simulink model "flight_data_collection"  (R2024a)
settings: Solver=FixedStepAuto  StartTime=0.0  StopTime=inf  FixedStep=0.1
model workspace (MAT data in the model file):
  Ixx_values = 1.545e-05
  Iyy_values = 0.00073574
  Izz_values = 0.00074861
  base_link_Ixx = 7.46
  base_link_Iyy = 1.52
  base_link_Izz = 8.88
  base_link_mass = 19.0939
  gps0_Ixx = 2.1733e-06
  gps0_Iyy = 2.1733e-06
  gps0_Izz = 1.8e-07
  gps0_mass = 0.01
  i = 8
  imu_link_Ixx = 1e-05
  imu_link_Iyy = 1e-05
  imu_link_Izz = 1e-05
  imu_link_mass = 0.015
  masses = 0.085251
  phi = sym
  phi.s = 'symobj::fromString("eJytVL1OwzAQdpqWPwkhoaJCp0jwBIydCoKBEYoYWCyHmGLkOCXnlGbjKXgneCpst6LONQ0MjfTJzt35u+/uLIeEkBYhH59mbYdBxyzDPpl/odl3F3sTQ3YtoAQGIMbKmSv+c4t3LvIkmrJcsFjySLGUQ1QATyKhIijTLH69KtK0vEm40uJZ8Jz4OVuIs23xksnE2HteTL9mj/W6syAzjexbFqATKWKXe48sv30L4HpUphdSMOAwr/PEy/HtxQeIe9tiAoI+MFvY8MzTebo84/79vAcWc02DwfVskpmO4Vl8efFt9N9BfE6Hx+P7QgujEfOv1EF/J13xHVmsHeWSs1M7jyIGpP2wQYebFeVvBZPkr3429crn3LGATE65uwGV3jjfJQPxNOIa8fRQrKsn51ZZhd/hjlZ6gTV1US2+77hulkJpPnYdXs31uLlcrv6caZGp+rpu6eYejP9epKZHofniCJXw2UpeVyQ1iZkC6j0sliP0mhFEixXbgzX2+8X6AxDlhOk=", 2)'
  phi.Digits = 32
  rotors(1).mass = 0.085251
  rotors(1).Ixx = 1.545e-05
  rotors(1).Iyy = 0.00073574
  rotors(1).Izz = 0.00074861
  rotors(2).mass = 0.085251
  rotors(2).Ixx = 1.545e-05
  rotors(2).Iyy = 0.00073574
  rotors(2).Izz = 0.00074861
  rotors(3).mass = 0.085251
  rotors(3).Ixx = 1.545e-05
  rotors(3).Iyy = 0.00073574
  rotors(3).Izz = 0.00074861
  rotors(4).mass = 0.085251
  rotors(4).Ixx = 1.545e-05
  rotors(4).Iyy = 0.00073574
  rotors(4).Izz = 0.00074861
  rotors(5).mass = 0.085251
  rotors(5).Ixx = 1.545e-05
  rotors(5).Iyy = 0.00073574
  rotors(5).Izz = 0.00074861
  rotors(6).mass = 0.085251
  rotors(6).Ixx = 1.545e-05
  rotors(6).Iyy = 0.00073574
  rotors(6).Izz = 0.00074861
  rotors(7).mass = 0.085251
  rotors(7).Ixx = 1.545e-05
  rotors(7).Iyy = 0.00073574
  rotors(7).Izz = 0.00074861
  rotors(8).mass = 0.085251
  rotors(8).Ixx = 1.545e-05
  rotors(8).Iyy = 0.00073574
  rotors(8).Izz = 0.00074861
  theta = sym
  theta.s = 'symobj::fromString("eJytVL1OwzAQdpqWPwkhoaJCp0jwBIydCoKBESoxsFgOOYqR45ScU5qNp+CdylNhuxV13DQwNNInO3fn7767sxwSQlqEfH7ptR0GHb0M+2TxhXrfXe51DNk3wBIZIh9La674Lw0+gOdJNGU5Z7GASLIUMCoQkojLCMs0i99uijQt7xKQir9wyImbs+Vxtg1eM5Foe8+J6dfsfb32LIpMefYdA1SJ4LHNfUBW36EBghqV6ZXgDAEXdZ45Ob6d+MDj3jWYIKePzBQ2vHB0nq/O2H8375HBQtNgcDubZLpj/izmTnzb++94fFaHw+P6QgOt0edfq4P+TrriOzHYOMoVZ6d2HkWMnvbjBh12VhTeCybIX/1s6pXLuWeAmZiCvQGV3ljfNUP+PALl8fS8WFtPDkZZhd/igVZ64WvqerW4vtO6WXKpYGw7vJ7raXu5bP05UzyT9XXd0+09GP+9SE2PQvPF4TKB2VpeWyTViZlE6jwshiN0mhFEy9W3BxvssFx/ABFthPo=", 2)'
  theta.Digits = 32
  total_Ixx = 7.46
  total_Iyy = 1.53
  total_Izz = 8.89
  total_mass = 20
  total_rotor_Ixx = 0.0001236
  total_rotor_Iyy = 0.00588592
  total_rotor_Izz = 0.00598888
  total_rotor_masses = 0.682008
  u = sym
  u.s = 'symobj::fromString("eJytVL1OwzAQdpqWPwkhoaJCp0jwBIydCoKBESoxsFgOOYqR45ScU5qNp+CdylNhuxV13DQwNNInO3fn7767sxwSQlqEfH7ptR0GHb0M+2TxhXrfXe51DNk3wBIZIh9La674Lw0+gOdJNGU5Z7GASLIUMCoQkojLCMs0i99uijQt7xKQir9wyImbs+Vxtg1eM5Foe8+J6dfsfb32LIpMefYdA1SJ4LHNfUBW36EBghqV6ZXgDAEXdZ45Ob6d+MDj3jWYIKePzBQ2vHB0nq/O2H8375HBQtNgcDubZLpj/izmTnzb++94fFaHw+P6QgOt0edfq4P+TrriOzHYOMoVZ6d2HkWMnvbjBh12VhTeCybIX/1s6pXLuWeAmZiCvQGV3ljfNUP+PALl8fS8WFtPDkZZhd/igVZ64WvqerW4vtO6WXKpYGw7vJ7raXu5bP05UzyT9XXd0+09GP+9SE2PQvPF4TKB2VpeWyTViZlE6jwshiN0mhFEy9W3Bxvs0+X6AxH1hQs=", 2)'
  u.Digits = 32
  v = sym
  v.s = 'symobj::fromString("eJytVL1OwzAQdpqWPwkhoaJCp0jwBIydCoKBESoxsFgOOYqR45ScU5qNjTfgneCpsN2KOm4aGBrpk52783ff3VkOCSEtQt4/9doOg45ehn0y/0K97y72OobsGmCJDJGPpTVX/OcGb8DzJJqynLNYQCRZChgVCEnEZYRlmsUvV0WaljcJSMWfOOTEzdnyONsGz5lItL3nxPRr9r5eexZFpjz7lgGqRPDY5t4jy2/fAEGNyvRCcIaA8zpPnBzfTnzgcW8bTJDTe2YKG545Ok+XZ+y/m/fAYK5pMLieTTLdMX8WX0582/vveHxWh8Pj+kIDrdHnX6mD/k664jsyWDvKJWendh5FjJ72wwYddlYUXgsmyF/9bOqVy7ljgJmYgr0Bld5Y3yVD/jgC5fH0vFhbTw5GWYXf4o5WeuFr6nq1uL7jullyqWBsO7ya62FzuWz9OVM8k/V13dLNPRj/vUhNj0LzxeEygdlKXlsk1YmZROo8LIYjdJoRRIvVtwdr7B+L9QcSfYUc", 2)'
  v.Digits = 32
  w = sym
  w.s = 'symobj::fromString("eJytVL1OwzAQdpqWPwkhoaJCp0jwBIydCoKBESoxsFgOOYqR45ScU5qNp0C8EjwVtltRx00DQyN9snN3/u67O8shIaRFyPuHXtth0NHLsE/mX6j33cVex5BdAyyRIfKxtOaK/9zgDXieRFOWcxYLiCRLAaMCIYm4jLBMs/jlqkjT8iYBqfgTh5y4OVseZ9vgOROJtvecmH7N3tdrz6LIlGffMkCVCB7b3Htk+e0bIKhRmV4IzhBwXueJk+PbiQ887m2DCXJ6z0xhwzNH5+nyjP138x4YzDUNBtezSaY75s/iy4lve/8dj8/qcHhcX2igNfr8K3XQ30lXfEcGa0e55OzUzqOI0dN+2KDDzorCa8EE+aufTb1yOXcMMBNTsDeg0hvru2TIH0egPJ6eF2vrycEoq/Bb3NFKL3xNXa8W13dcN0suFYxth1dzPWwul60/Z4pnsr6uW7q5B+O/F6npUWi+OFwmMFvJa4ukOjGTSJ2HxXCETjOCaLH69mCN/XOx/gATBYUt", 2)'
  w.Digits = 32
  x = sym
  x.s = 'symobj::fromString("eJytVEtOwzAQdZqWn4SQUFGhq0hwApZdFQQLllCJBRvLIUMxcpyScUqz4xTcgaPAqbDdijpuGlg00pOdmfGbNzOWQ0JIi5D3D722w6Cjl2GfzL9Q77uLvY4huwZYIkPkY2nNFf+5wRvwPImmLOcsFhBJlgJGBUIScRlhmWbxy1WRpuVNAlLxJw45cXO2PM62wXMmEm3vOTH9mr2v155FkSnPvmWAKhE8trn3yPLbN0BQozK9EJwh4LzOEyfHtxMfeNzbBhPk9J6ZwoZnjs7T5Rn77+Y9MJhrGgyuZ5NMd8yfxZcT3/b+Ox6f1eHwuL7QQGv0+VfqoL+TrviODNaOcsnZqZ1HEaOn/bBBh50VhdeCCfJXP5t65XLuGGAmpmBvQKU31nfJkD+OQHk8PS/W1pODUVbht7ijlV74mrpeLa7vuG6WXCoY2w6v5nrYXC5bf84Uz2R9Xbd0cw/Gfy9S06PQfHG4TGC2ktcWSXViJpE6D4vhCJ1mBNFi9e3BGvvnYv0BE42FPg==", 2)'
  x.Digits = 32
  y = sym
  y.s = 'symobj::fromString("eJytVEtOwzAQdZqWn4SQUFGhq0hwApZdFQQLllCJBRvLIUMxcpyScUqz4xQchhvAqbDdijpuGlg00pOdmfGbNzOWQ0JIi5D3D722w6Cjl2GfzL9Q77uLvY4huwZYIkPkY2nNFf+5wRvwPImmLOcsFhBJlgJGBUIScRlhmWbxy1WRpuVNAlLxJw45cXO2PM62wXMmEm3vOTH9mr2v155FkSnPvmWAKhE8trn3yPLbN0BQozK9EJwh4LzOEyfHtxMfeNzbBhPk9J6ZwoZnjs7T5Rn77+Y9MJhrGgyuZ5NMd8yfxZcT3/b+Ox6f1eHwuL7QQGv0+VfqoL+TrviODNaOcsnZqZ1HEaOn/bBBh50VhdeCCfJXP5t65XLuGGAmpmBvQKU31nfJkD+OQHk8PS/W1pODUVbht7ijlV74mrpeLa7vuG6WXCoY2w6v5nrYXC5bf84Uz2R9Xbd0cw/Gfy9S06PQfHG4TGC2ktcWSXViJpE6D4vhCJ1mBNFi9e3BGvvnYv0BFBWFTw==", 2)'
  y.Digits = 32
  z = sym
  z.s = 'symobj::fromString("eJytVL1OwzAQdpqWPwkhoaJCp0jwBIydCoKBESoxsFgOOYqR45ScU5qNp+CdgJfCdivquGlgaKRPdu7O3313ZzkkhLQIef/QazsMOnoZ9sn8C/W+u9jrGLJrgCUyRD6W1lzxnxu8Ac+TaMpyzmIBkWQpYFQgJBGXEZZpFr9cFWla3iQgFX/ikBM3Z8vjbBs8ZyLR9p4T06/Z+3rtWRSZ8uxbBqgSwWObe48sv30DBDUq0wvBGQLO6zxxcnw58YHHvW0wQU7vmSlseOboPF2esf9u3gODuabB4Ho2yXTH/Fl8OvFt77/j8VkdDo/rCw20Rp9/pQ76O+mK78hg7SiXnJ3aeRQxetoPG3TYWVF4LZggf/WzqVcu544BZmIK9gZUemN9lwz54wiUx9PzYm09ORhlFX6LO1rpha+p69Xi+o7rZsmlgrHt8Gquh83lsvXnTPFM1td1Szf3YPz3IjU9Cs0Xh8sEZit5bZFUJ2YSqfOwGI7QaUYQLVbfHqyxfy/WHxSdhWA=", 2)'
  z.Digits = 32
undefined symbols (not defined in the file or in its folder): rad, s
libraries: robotlib x15, simulink x3, eeGeneralControl x3, aerolibconvert2 x1, sharedtransform x1
settings Model: PacingRate=100  Creator=hmcl  LastModifiedBy=hmcl
settings OptimizationCC: EnhancedBackFolding=on  PassReuseOutputArgsAs=Individual arguments  ZeroExternalMemoryAtStartup=off  ZeroInternalMemoryAtStartup=off  MaxStackSize=64  OptimizeBlockOrder=speed  DifferentSizesBufferReuse=on  OptimizationCustomize=off  EfficientTunableParamExpr=on
settings DebuggingCC: ParameterTunabilityLossMsg=error
settings HardwareCC: ProdBitPerPointer=32  ProdBitPerSizeT=32  ProdBitPerPtrDiffT=32  ProdLargestAtomicFloat=None  ProdIntDivRoundTo=Undefined  ProdEndianess=Unspecified  ProdWordSize=32  ProdHWDeviceType=Generic->Unspecified (assume 32-bit Generic)
settings SFSimCC: MATLABDynamicMemAlloc=off
settings RTWCC: Description=Embedded Coder  SystemTargetFile=ert.tlc  HardwareBoard=Robot Operating System (ROS)  TLCOptions="-aInlineSetEventsForThisBaseRateFcn=TLC_FALSE -aSuppressMultiTaskScheduler=TLC_FALSE  -aRateBasedStepFcn=0"  TemplateMakefile=ert_default_tmf  Toolchain=Catkin  TargetLang=C++  GPUComputeCapability=3.5
settings CodeAppCC: ForceParamTrailComments=on  IgnoreCustomStorageClasses=off  OperatorAnnotations=on  SimulinkDataObjDesc=on  SFDataObjDesc=on  InsertBlockDesc=on
settings ERTTargetCC: CodeInterfacePackaging=C++ class  RootIOFormat=Structure reference

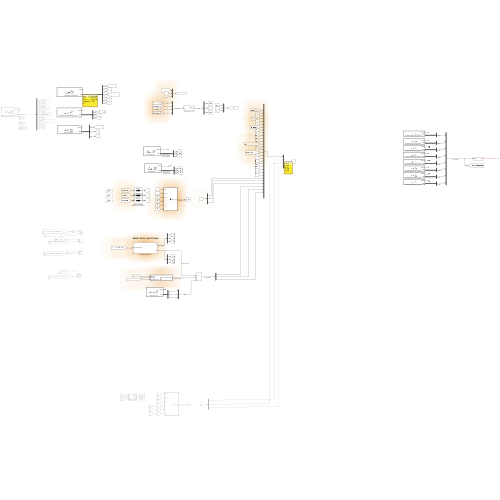
[thumbnail: Simulink's stored preview of the top-level diagram]
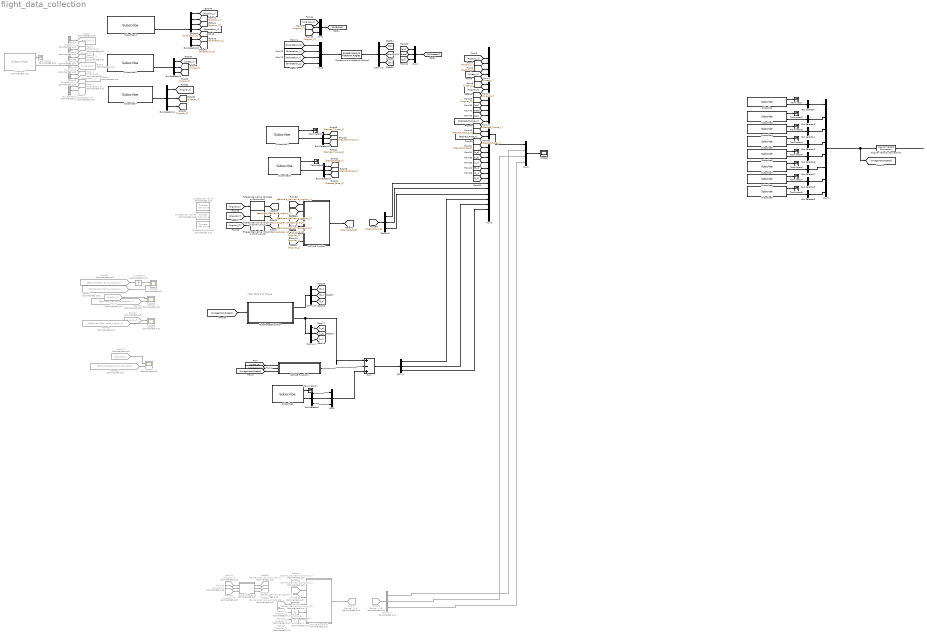
== system flight_data_collection ==
  note: Motor Force and Torque
  Angular Velocity Conversion1 : aerolibconvert2/Angular Velocity Conversion  IU=rad/s  OU=rpm
  Bus Selector{,3..9} (8 alike) : BusSelector  OutputSignals=Data
  Bus Selector1 : BusSelector  Commented=on  OutputSignals=Pose.Pose.Position.X,Pose.Pose.Position.Y,Pose.Pose.Position.Z,Twist.Twist.Linear.X,Twist.Twist.Linear.Y,Twist.Twist.Linear.Z,Twist.Twist.Angular.X,Twist.Twist.Angular.Y,Twist.Twist.Angular.Z,Pose.Pose.Orientation.X,Pose.Pose.Orientation.Y,Pose.Pose.Orientation.Z,Pose.Pose.Orientation.W
  Bus Selector10 : BusSelector  OutputSignals=X,Y,Z
  Bus Selector11 : BusSelector  OutputSignals=X,Y,Z
  Bus Selector12 : BusSelector  OutputSignals=Pose.Position.X,Pose.Position.Y,Pose.Position.Z,Pose.Orientation.X,Pose.Orientation.Y,Pose.Orientation.Z,Pose.Orientation.W
  Bus Selector13 : BusSelector  OutputSignals=Twist.Linear.X,Twist.Linear.Y,Twist.Linear.Z
  Bus Selector14 : BusSelector  OutputSignals=AngularVelocity.X,AngularVelocity.Y,AngularVelocity.Z
  Bus Selector2 : BusSelector  OutputSignals=X,Y,Z
  Demux{,2..5} (5 alike) : Demux  Outputs=3
  Demux1 : Demux  Commented=on  Outputs=3
  Discrete Derivative : simulink/Discrete/Discrete Derivative  Commented=on  gainval=1  ICPrevScaledInput=0.0  OutMin=[]  OutMax=[]  OutDataType=fixdt(1, 16)  OutScaling=2^-10  DoSatur=off
  Discrete Derivative1 : simulink/Discrete/Discrete Derivative  Commented=on  gainval=1  ICPrevScaledInput=0.0  OutMin=[]  OutMax=[]  OutDataType=fixdt(1, 16)  OutScaling=2^-10  DoSatur=off
  Discrete Derivative2 : simulink/Discrete/Discrete Derivative  Commented=on  gainval=1  ICPrevScaledInput=0.0  OutMin=[]  OutMax=[]  OutDataType=fixdt(1, 16)  OutScaling=2^-10  DoSatur=off
  Filtered Derivative (Discrete or Continuous) : eeGeneralControl/Filtered Derivative (Discrete or Continuous)  K=1  T=0.01  B=inf  A=-inf  minRatio=10  init_option=Inherited from block input  x0=0  Ts=-1
      settings: LibrarySourceBlock=|
      | ee_sl_lib/General Control/Filtered Derivative
      | (Discrete or Continuous)
  Filtered Derivative (Discrete or Continuous)1 : eeGeneralControl/Filtered Derivative (Discrete or Continuous)  K=1  T=0.01  B=inf  A=-inf  minRatio=10  init_option=Inherited from block input  x0=0  Ts=-1
      settings: LibrarySourceBlock=|
      | ee_sl_lib/General Control/Filtered Derivative
      | (Discrete or Continuous)
  Filtered Derivative (Discrete or Continuous)2 : eeGeneralControl/Filtered Derivative (Discrete or Continuous)  K=1  T=0.01  B=inf  A=-inf  minRatio=10  init_option=Inherited from block input  x0=0  Ts=-1
      settings: LibrarySourceBlock=|
      | ee_sl_lib/General Control/Filtered Derivative
      | (Discrete or Continuous)
  From10 : From  Commented=on  GotoTag=Angular_X
  From11 : From  Commented=on  GotoTag=Angular_X
  From18 : From  Commented=on  GotoTag=Angular_Y
  From21 : From  Commented=on  GotoTag=Angular_Y
  From24 : From  Commented=on  GotoTag=Angular_Y
  From27 : From  Commented=on  GotoTag=Angular_Z
  From32 : From  Commented=on  GotoTag=Angular_Z
  From33 : From  Commented=on  GotoTag=Angular_Z
  From57 : From  Commented=on  GotoTag=Backward_Derivative_Angular_X
  From58 : From  Commented=on  GotoTag=Backward_Derivative_Angular_X
  From60 : From  Commented=on  GotoTag=Backward_Derivative_Angular_Y
  From62 : From  Commented=on  GotoTag=Backward_Derivative_Angular_Z
  From63 : From  Commented=on  GotoTag=Central_Derivative_Angular_X
  From64 : From  Commented=on  GotoTag=Central_Derivative_Angular_X
  From65 : From  Commented=on  GotoTag=Central_Derivative_Angular_Y
  From66 : From  Commented=on  GotoTag=Central_Derivative_Angular_Z
  From70 : From  Commented=on  GotoTag=Central_M_B
  From9 : From  Commented=on  GotoTag=Angular_X
  Goto10 : Goto  Commented=on  GotoTag=Angular_Y
  Goto11 : Goto  Commented=on  GotoTag=Angular_Z
  Goto12 : Goto  Commented=on  GotoTag=Orientation_X
  Goto13 : Goto  Commented=on  GotoTag=Orientation_Y
  Goto14 : Goto  Commented=on  GotoTag=Orientation_Z
  Goto15 : Goto  Commented=on  GotoTag=Orientation_W
  Goto28 : Goto  Commented=on  GotoTag=Central_Derivative_Angular_X
  Goto29 : Goto  Commented=on  GotoTag=Central_Derivative_Angular_Y
  Goto3 : Goto  Commented=on  GotoTag=Position_X
  Goto30 : Goto  Commented=on  GotoTag=Central_Derivative_Angular_Z
  Goto32 : Goto  Commented=on  GotoTag=Central_M_B
  Goto4 : Goto  Commented=on  GotoTag=Position_Y
  Goto5 : Goto  Commented=on  GotoTag=Position_Z
  Goto6 : Goto  Commented=on  GotoTag=Linear_X
  Goto7 : Goto  Commented=on  GotoTag=Linear_Y
  Goto8 : Goto  Commented=on  GotoTag=Linear_Z
  Goto9 : Goto  Commented=on  GotoTag=Angular_X
  MATLAB Function : MATLAB Function  TreatAsAtomicUnit=on
  MATLAB Function1 : MATLAB Function  TreatAsAtomicUnit=on
  MATLAB Function3 : MATLAB Function  Commented=on  TreatAsAtomicUnit=on
  MotorForceCalculation : Subsystem  mask{Ct=-0.00053, Cq=0.0000169, L1=0.545, L2=0.36, L3=1.08}
      mask prompts: Ct "Ct = motorConstant [N*s^2/rad^2] ="; Cq "Cq = momentConstant [N*m*s^2/rad^2] ="; L1 "L1 ="; L2 "L2 ="; L3 "L3 ="
  Mux1 : Mux  Inputs=3
  Mux2 : Mux  Inputs=3
  Mux3 : Mux  Inputs=3
  Mux5 : Mux  Inputs=30
  Mux6 : Mux
  Mux8 : Mux
  Mux9 : Mux  Inputs=8
  Quaternions to Rotation Angles1 : sharedtransform/Quaternions to Rotation Angles  rotationOrder=ZYX  aMode=aMode
  Scope{1,5..7} (4 alike) : Scope  Commented=on  NumInputPorts=2
  Scope2 : Scope
  Subscribe : robotlib/Subscribe  topicSource=Select from ROS network  topic=/my/octocopter3/motor_speed/0  messageType=std_msgs/Float64  SampleTime=-1  legacyBusStruct=off  messageQueueLength=1
  Subscribe1 : robotlib/Subscribe  Commented=on  topicSource=Select from ROS network  topic=/mavros/local_position/odom  messageType=nav_msgs/Odometry  SampleTime=-1  legacyBusStruct=off  messageQueueLength=1
  Subscribe10 : robotlib/Subscribe  topicSource=Select from ROS network  topic=/thrust_vector  messageType=geometry_msgs/Vector3  SampleTime=-1  legacyBusStruct=off  messageQueueLength=1
  Subscribe11 : robotlib/Subscribe  topicSource=Select from ROS network  topic=/torque_vector  messageType=geometry_msgs/Vector3  SampleTime=-1  legacyBusStruct=off  messageQueueLength=1
  Subscribe12 : robotlib/Subscribe  topicSource=Select from ROS network  topic=/mavros/local_position/pose  messageType=geometry_msgs/PoseStamped  SampleTime=-1  legacyBusStruct=off  messageQueueLength=1
  Subscribe13 : robotlib/Subscribe  topicSource=Select from ROS network  topic=/mavros/local_position/velocity_local  messageType=geometry_msgs/TwistStamped  SampleTime=-1  legacyBusStruct=off  messageQueueLength=1
  Subscribe14 : robotlib/Subscribe  topicSource=Select from ROS network  topic=/mavros/imu/data  messageType=sensor_msgs/Imu  SampleTime=-1  legacyBusStruct=off  messageQueueLength=1
  Subscribe2 : robotlib/Subscribe  topicSource=Select from ROS network  topic=/wind_gust_pub  messageType=geometry_msgs/Vector3  SampleTime=-1  legacyBusStruct=off  messageQueueLength=1
  Subscribe3 : robotlib/Subscribe  topicSource=Select from ROS network  topic=/my/octocopter3/motor_speed/1  messageType=std_msgs/Float64  SampleTime=-1  legacyBusStruct=off  messageQueueLength=1
  Subscribe4 : robotlib/Subscribe  topicSource=Select from ROS network  topic=/my/octocopter3/motor_speed/2  messageType=std_msgs/Float64  SampleTime=-1  legacyBusStruct=off  messageQueueLength=1
  Subscribe5 : robotlib/Subscribe  topicSource=Select from ROS network  topic=/my/octocopter3/motor_speed/3  messageType=std_msgs/Float64  SampleTime=-1  legacyBusStruct=off  messageQueueLength=1
  Subscribe6 : robotlib/Subscribe  topicSource=Select from ROS network  topic=/my/octocopter3/motor_speed/4  messageType=std_msgs/Float64  SampleTime=-1  legacyBusStruct=off  messageQueueLength=1
  Subscribe7 : robotlib/Subscribe  topicSource=Select from ROS network  topic=/my/octocopter3/motor_speed/5  messageType=std_msgs/Float64  SampleTime=-1  legacyBusStruct=off  messageQueueLength=1
  Subscribe8 : robotlib/Subscribe  topicSource=Select from ROS network  topic=/my/octocopter3/motor_speed/6  messageType=std_msgs/Float64  SampleTime=-1  legacyBusStruct=off  messageQueueLength=1
  Subscribe9 : robotlib/Subscribe  topicSource=Select from ROS network  topic=/my/octocopter3/motor_speed/7  messageType=std_msgs/Float64  SampleTime=-1  legacyBusStruct=off  messageQueueLength=1
  Sum : Sum  Inputs=|+-+
  Terminator{,2..11} (11 alike) : Terminator
  Terminator1 : Terminator  Commented=on
  Unit Delay{,1..2,5} (4 alike) : UnitDelay  Commented=on  SampleTime=-1  HasFrameUpgradeWarning=on
  central difference : MATLAB Function  Commented=on  TreatAsAtomicUnit=on
  wires:
  Subscribe1/2 -> Bus Selector1/1  "Position_X = x  Position_Y = y Position_Z = z Linear_X = u Linear_Y = v Linear_Z = w Angular_X = p Angular_Y = q Angular_Z = r Orientation_X = q1  Orientation_Y = q2 Orientation_Z = q3 Orientation_W = q4"
  Subscribe1/1 -> Terminator1/1
  Subscribe/1 -> Terminator/1
  Subscribe3/1 -> Terminator2/1
  Subscribe4/1 -> Terminator3/1
  Subscribe5/1 -> Terminator4/1
  Subscribe6/1 -> Terminator5/1
  Subscribe7/1 -> Terminator6/1
  Subscribe8/1 -> Terminator7/1
  Subscribe9/1 -> Terminator8/1
  Subscribe/2 -> Bus Selector/1
  Subscribe3/2 -> Bus Selector3/1
  Subscribe4/2 -> Bus Selector4/1
  Subscribe5/2 -> Bus Selector5/1
  Subscribe6/2 -> Bus Selector6/1
  Subscribe7/2 -> Bus Selector7/1
  Subscribe8/2 -> Bus Selector8/1
  Subscribe9/2 -> Bus Selector9/1
  Mux9/1 -> Angular Velocity Conversion1/1, [omegaMotorSpeed]  "motorSpeed"
  Bus Selector/1 -> Mux9/1  "<Data>"
  Bus Selector3/1 -> Mux9/2  "<Data>"
  Bus Selector4/1 -> Mux9/3  "<Data>"
  Bus Selector5/1 -> Mux9/4  "<Data>"
  Bus Selector6/1 -> Mux9/5  "<Data>"
  Bus Selector7/1 -> Mux9/6  "<Data>"
  Bus Selector8/1 -> Mux9/7  "<Data>"
  Bus Selector9/1 -> Mux9/8  "<Data>"
  Angular Velocity Conversion1/1 -> ?
  Subscribe10/1 -> Terminator9/1
  Subscribe11/1 -> Terminator10/1
  Subscribe10/2 -> Bus Selector10/1  "Desired_Force_X Desired_Force_Y Desired_Force_Z"
  Subscribe11/2 -> Bus Selector11/1  "Desired_Torque_X Desired_Torque_Y Desired_Torque_Z"
  Demux5/1 -> Mux5/25
  Demux5/2 -> Mux5/26
  Demux5/3 -> Mux5/27
  [omegaMotorSpeed] -> MotorForceCalculation/1(omegaMotorSpeed)
  [OMEGAB] -> MATLAB Function1/1(OMEGA_B)
  Mux2/1 -> [phithetapsi]
  [phithetapsi] -> MATLAB Function1/2(phithetapsi)
  [omegaMotorSpeed] -> MATLAB Function1/3(omegaMotorSpeed)
  Subscribe2/1 -> Terminator11/1
  Subscribe2/2 -> Bus Selector2/1
  MATLAB Function1/1(gyroscopic_effect) -> Sum/2
  MotorForceCalculation/2(MB) -> Demux4/1, Sum/1  "moment on body"
  Bus Selector2/1 -> Mux3/1  "<X>"
  Bus Selector2/2 -> Mux3/2  "<Y>"
  Bus Selector2/3 -> Mux3/3  "<Z>"
  Mux3/1 -> Sum/3  "wind"
  MotorForceCalculation/1(FB) -> Demux3/1  "force on body"
  Unit Delay/1 -> MATLAB Function3/4(p)
  Unit Delay1/1 -> MATLAB Function3/5(q)
  Unit Delay2/1 -> MATLAB Function3/6(r)
  Unit Delay5/1 -> Scope5/1
  Sum/1 -> Demux/1  "nominal MB"
  Demux/1 -> Mux5/28
  Demux/2 -> Mux5/29
  Demux/3 -> Mux5/30
  Mux5/1 -> Mux6/1
  Mux6/1 -> Scope2/1
  Demux1/1 -> Mux6/2
  Demux1/2 -> Mux6/3
  Demux1/3 -> Mux6/4
  Bus Selector1/1 -> Goto3/1  "<X>"
  [Position_X] -> Mux5/1
  Bus Selector1/2 -> Goto4/1  "<Y>"
  [Position_Y] -> Mux5/2
  Bus Selector1/3 -> Goto5/1  "<Z>"
  [Position_Z] -> Mux5/3
  Bus Selector1/4 -> Goto6/1  "<X>"
  [Linear_X] -> Mux5/4
  Bus Selector1/5 -> Goto7/1  "<Y>"
  [Linear_Y] -> Mux5/5
  Bus Selector1/6 -> Goto8/1  "<Z>"
  [Linear_Z] -> Mux5/6
  Bus Selector1/7 -> Goto9/1  "<X>"
  From9/1 -> Scope1/1
  From10/1 -> central difference/1(p)
  From11/1 -> Unit Delay/1
  [Angular_X] -> Mux5/7
  [Angular_X] -> MATLAB Function/4(p)
  Bus Selector1/8 -> Goto10/1  "<Y>"
  [Angular_Y] -> Filtered Derivative (Discrete or Continuous)1/1
  From18/1 -> Scope6/1
  [Angular_Y] -> MATLAB Function/5(q)
  From21/1 -> Unit Delay1/1
  [Angular_Y] -> Mux5/8
  From24/1 -> central difference/2(q)
  Bus Selector1/9 -> Goto11/1  "<Z>"
  [Angular_Z] -> Filtered Derivative (Discrete or Continuous)2/1
  From27/1 -> Scope7/1
  [Angular_Z] -> Mux5/9
  [Angular_Z] -> MATLAB Function/6(r)
  From32/1 -> central difference/3(r)
  From33/1 -> Unit Delay2/1
  Bus Selector1/10 -> Goto12/1  "<X>"
  Bus Selector1/11 -> Goto13/1  "<Y>"
  Bus Selector1/12 -> Goto14/1  "<Z>"
  Bus Selector1/13 -> Goto15/1  "<W>"
  [phi] -> Mux5/10
  [phi] -> Mux2/1
  [theta] -> Mux5/11
  [theta] -> Mux2/2
  [psi] -> Mux2/3
  [psi] -> Mux5/12
  Bus Selector11/1 -> [Desired_Torque_X]  "<X>"
  [Desired_Torque_X] -> Mux5/13
  Bus Selector11/2 -> [Desired_Torque_Y]  "<Y>"
  [Desired_Torque_Y] -> Mux5/14
  Bus Selector11/3 -> [Desired_Torque_Z]  "<Z>"
  [Desired_Torque_Z] -> Mux5/15
  Bus Selector10/1 -> [Desired_Force_X]  "<X>"
  [Desired_Force_X] -> Mux5/16
  Bus Selector10/2 -> [Desired_Force_Y]  "<Y>"
  [Desired_Force_Y] -> Mux5/17
  Bus Selector10/3 -> [Desired_Force_Z]  "<Z>"
  [Desired_Force_Z] -> Mux5/18
  Filtered Derivative (Discrete or Continuous)/1 -> [Backward_Derivative_Angular_X]
  [Backward_Derivative_Angular_X] -> MATLAB Function/1(p_dot)
  From57/1 -> Unit Delay5/1
  From58/1 -> Scope1/2
  Filtered Derivative (Discrete or Continuous)1/1 -> [Backward_Derivative_Angular_Y]
  [Backward_Derivative_Angular_Y] -> MATLAB Function/2(q_dot)
  From60/1 -> Scope6/2
  Filtered Derivative (Discrete or Continuous)2/1 -> [Backward_Derivative_Angular_Z]
  [Backward_Derivative_Angular_Z] -> MATLAB Function/3(r_dot)
  From62/1 -> Scope7/2
  central difference/1(p_dot) -> Goto28/1
  From63/1 -> Scope5/2
  From64/1 -> MATLAB Function3/1(p_dot)
  central difference/2(q_dot) -> Goto29/1
  From65/1 -> MATLAB Function3/2(q_dot)
  central difference/3(r_dot) -> Goto30/1
  From66/1 -> MATLAB Function3/3(r_dot)
  MATLAB Function/1(backward_M_B) -> [backward_M_B]  "backward_M_B"
  [backward_M_B] -> Demux5/1
  MATLAB Function3/1(Central_M_B) -> Goto32/1  "Central_M_B"
  From70/1 -> Demux1/1
  Demux2/3 -> [phi]
  Quaternions to Rotation Angles1/1 -> Demux2/1  "radian"
  [Orientation_Z] -> Mux8/4  "z"
  Demux2/2 -> [theta]
  [Orientation_X] -> Mux8/2  "x"
  [Orientation_Y] -> Mux8/3  "Y"
  [Orientation_W] -> Mux8/1  "W"
  Mux8/1 -> Quaternions to Rotation Angles1/1  "quertanion"
  Demux2/1 -> [psi]
  Mux1/1 -> [OMEGAB]
  [Angular_X] -> Mux1/1
  [Angular_Y] -> Mux1/2
  [Angular_Z] -> Mux1/3
  Demux4/1 -> [u_p]
  Demux4/2 -> [u_q]
  Demux4/3 -> [u_r]
  Demux3/2 -> [f_y]
  Demux3/3 -> [f_z]
  Demux3/1 -> [f_x]
  [u_p] -> Mux5/19
  [u_q] -> Mux5/20
  [u_r] -> Mux5/21
  [f_x] -> Mux5/22
  [f_y] -> Mux5/23
  [f_z] -> Mux5/24
  [Angular_X] -> Filtered Derivative (Discrete or Continuous)/1
  Subscribe12/2 -> Bus Selector12/1
  Bus Selector12/1 -> [Position_X]  "<X>"
  Bus Selector12/2 -> [Position_Y]  "<Y>"
  Bus Selector12/3 -> [Position_Z]  "<Z>"
  Bus Selector12/4 -> [Orientation_X]  "<X>"
  Bus Selector12/5 -> [Orientation_Y]  "<Y>"
  Bus Selector12/6 -> [Orientation_Z]  "<Z>"
  Bus Selector12/7 -> [Orientation_W]  "<W>"
  Subscribe13/2 -> Bus Selector13/1
  Bus Selector13/1 -> [Linear_X]  "<X>"
  Bus Selector13/2 -> [Linear_Y]  "<Y>"
  Bus Selector13/3 -> [Linear_Z]  "<Z>"
  Subscribe14/2 -> Bus Selector14/1
  Bus Selector14/3 -> [Angular_Z]  "<Z>"
  Bus Selector14/2 -> [Angular_Y]  "<Y>"
  Bus Selector14/1 -> [Angular_X]  "<X>"

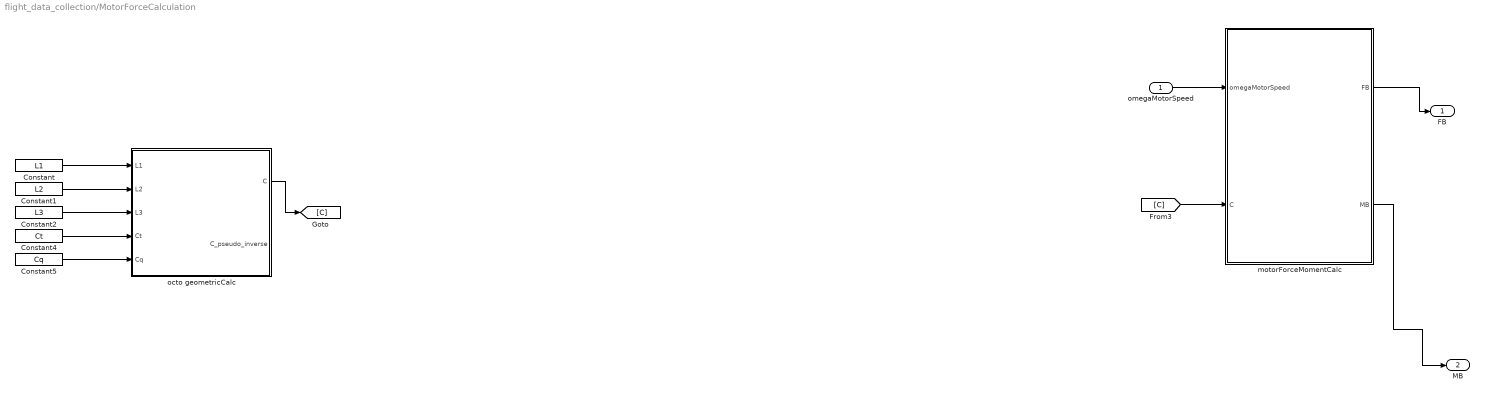
== system flight_data_collection/MotorForceCalculation ==
  omegaMotorSpeed : Inport
  Constant : Constant  Value=L1
  Constant1 : Constant  Value=L2
  Constant2 : Constant  Value=L3
  Constant4 : Constant  Value=Ct
  Constant5 : Constant  Value=Cq
  motorForceMomentCalc : MATLAB Function  TreatAsAtomicUnit=on
  octo geometricCalc : MATLAB Function  TreatAsAtomicUnit=on
  FB : Outport
  MB : Outport  Port=2
  wires:
  motorForceMomentCalc/1(FB) -> FB/1
  motorForceMomentCalc/2(MB) -> MB/1
  [C] -> motorForceMomentCalc/2(C)
  omegaMotorSpeed/1 -> motorForceMomentCalc/1(omegaMotorSpeed)
  Constant5/1 -> octo geometricCalc/5(Cq)
  Constant2/1 -> octo geometricCalc/3(L3)
  Constant4/1 -> octo geometricCalc/4(Ct)
  Constant/1 -> octo geometricCalc/1(L1)
  Constant1/1 -> octo geometricCalc/2(L2)
  octo geometricCalc/1(C) -> [C]

== matlab function flight_data_collection/MATLAB Function1 ==
  data: gyroscopic_effect output; OMEGA_B input; phithetapsi input; omegaMotorSpeed input
function gyroscopic_effect = fcn(OMEGA_B, phithetapsi, omegaMotorSpeed)

% coder.extrinsic('RotMat');
% coder.extrinsic('cross');
% coder.extrinsic('size');

% OMEGA_B : 3by1
p = OMEGA_B(1);
q = OMEGA_B(2);
r = OMEGA_B(3);
% disp('OMEGA_B = ');
% disp(size(OMEGA_B))

phi = phithetapsi(1);
theta = phithetapsi(2);
psi = phithetapsi(3);

ga = zeros(3, 1); % 각 로터에 대한 자이로스코픽 모멘트 저장
e_z_hat = [0;0;1]; % 가제보 좌표를 기반으로 z축의 unit vector
J_p = [1.545e-05 0 0;0 7.3574e-04 0;0 0 7.4861e-04]; % the moment of inertia related to 3 axes of body frame
% J_p = [0.001 0 0;0 0.001 0;0 0 0.006];

% e_z_hat : the unit vector in the inertial z axis
% e_3_hat : the unit vector in the body z axis : 3by1
e_3_hat = RotMat(phi, theta, psi, 8) * e_z_hat;  


% 부호 배열 (로터 방향에 따른 부호), Cq의 부호 사용
signs = [1; 1; -1; -1; -1; -1; 1; 1];

% 자이로스코픽 효과 계산
% cross(OMEGA_B, e_3_hat) : 3by1
% sum(signs .* abs(omegaMotorSpeed)) : 1by1
% ga : 3by1
ga = J_p * cross(OMEGA_B, e_3_hat) * sum(signs .* abs(omegaMotorSpeed));
gyroscopic_effect = ga;

end



%%
function rm = RotMat(phi, theta, psi, int)

% Module for transforming the p vector from one frame to another frame
% Possible transformations
% 1 - Transformation from the inertial frame (i - North, j - East, k - Towards earth center) to vehicle frame 1
% 2 - Transformation from the vehicle frame 1 to vehicle frame 2
% 3 - Transformation from the vehicle frame 2 to body frame
% 4 - Transformation from the vehicle frame (inertial frame) to body frame
% 5 - Transformation from the body frame to vehicle frame (inertial frame)
% 6 - Transformation from the derivative of (phi theta psi) to body rates (p q r)
% 7 - Transformation from the body rates (p q r) to derivative of (phi theta psi)

switch int

    case 1  %Rz                                                               % Transformation from vehicle frame (i - North, j - East, k - Towards earth center) to vehicle frame 1

        rm = [ cos(psi)     sin(psi)       0  ;
            -sin(psi)     cos(psi)       0  ;
            0             0           1 ];

    case 2  %Ry                                                               % Transformation from vehicle frame 1 to vehicle frame 2

        rm = [ cos(theta)    0       -sin(theta)  ;
            0          1            0       ;
            sin(theta)    0        cos(theta) ];

    case 3     %Rx                                                            % Transformation from vehicle frame 2 to body frame
        rm = [ 1              0             0      ;
            0            cos(phi)     sin(phi)  ;
            0           -sin(phi)     cos(phi) ];

    case 4       %inv(R)                                                          
        rm = [
            (cos(psi)*cos(theta))/(cos(psi)^2*cos(theta)^2 + cos(psi)^2*sin(theta)^2 + cos(theta)^2*sin(psi)^2 + sin(psi)^2*sin(theta)^2), ...
            (cos(theta)*sin(psi))/(cos(psi)^2*cos(theta)^2 + cos(psi)^2*sin(theta)^2 + cos(theta)^2*sin(psi)^2 + sin(psi)^2*sin(theta)^2), ...
            -sin(theta)/(cos(theta)^2 + sin(theta)^2);

            -(cos(phi)*cos(theta)^2*sin(psi) + cos(phi)*sin(psi)*sin(theta)^2 - cos(psi)*sin(phi)*sin(theta))/(cos(phi)^2*cos(psi)^2*sin(theta)^2 + cos(phi)^2*cos(theta)^2*sin(psi)^2 + cos(psi)^2*cos(theta)^2*sin(phi)^2 + cos(phi)^2*sin(psi)^2*sin(theta)^2 + cos(psi)^2*sin(phi)^2*sin(theta)^2 + cos(theta)^2*sin(phi)^2*sin(psi)^2 + sin(phi)^2*sin(psi)^2*sin(theta)^2 + cos(phi)^2*cos(psi)^2*cos(theta)^2), ...
            (sin(phi)*sin(psi)*sin(theta) + cos(phi)*cos(psi)*cos(theta)^2 + cos(phi)*cos(psi)*sin(theta)^2)/(cos(phi)^2*cos(psi)^2*sin(theta)^2 + cos(phi)^2*cos(theta)^2*sin(psi)^2 + cos(psi)^2*cos(theta)^2*sin(phi)^2 + cos(phi)^2*sin(psi)^2*sin(theta)^2 + cos(psi)^2*sin(phi)^2*sin(theta)^2 + cos(theta)^2*sin(phi)^2*sin(psi)^2 + sin(phi)^2*sin(psi)^2*sin(theta)^2 + cos(phi)^2*cos(psi)^2*cos(theta)^2), ...
            (cos(theta)*sin(phi))/(cos(phi)^2*cos(theta)^2 + cos(phi)^2*sin(theta)^2 + cos(theta)^2*sin(phi)^2 + sin(phi)^2*sin(theta)^2);

            (cos(theta)^2*sin(phi)*sin(psi) + sin(phi)*sin(psi)*sin(theta)^2 + cos(phi)*cos(psi)*sin(theta))/(cos(phi)^2*cos(psi)^2*sin(theta)^2 + cos(phi)^2*cos(theta)^2*sin(psi)^2 + cos(psi)^2*cos(theta)^2*sin(phi)^2 + cos(phi)^2*sin(psi)^2*sin(theta)^2 + cos(psi)^2*sin(phi)^2*sin(theta)^2 + cos(theta)^2*sin(phi)^2*sin(psi)^2 + sin(phi)^2*sin(psi)^2*sin(theta)^2 + cos(phi)^2*cos(psi)^2*cos(theta)^2), ...
            -(cos(psi)*cos(theta)^2*sin(phi) + cos(psi)*sin(phi)*sin(theta)^2 - cos(phi)*sin(psi)*sin(theta))/(cos(phi)^2*cos(psi)^2*sin(theta)^2 + cos(phi)^2*cos(theta)^2*sin(psi)^2 + cos(psi)^2*cos(theta)^2*sin(phi)^2 + cos(phi)^2*sin(psi)^2*sin(theta)^2 + cos(psi)^2*sin(phi)^2*sin(theta)^2 + cos(theta)^2*sin(phi)^2*sin(psi)^2 + sin(phi)^2*sin(psi)^2*sin(theta)^2 + cos(phi)^2*cos(psi)^2*cos(theta)^2), ...
            (cos(phi)*cos(theta))/(cos(phi)^2*cos(theta)^2 + cos(phi)^2*sin(theta)^2 + cos(theta)^2*sin(phi)^2 + sin(phi)^2*sin(theta)^2)
            ];


    case 5     %R                                                            % Transformation from body frame to inertial frame
        rm = [cos(psi)*cos(theta), cos(psi)*sin(theta)*sin(phi) - sin(psi)*cos(phi), cos(psi)*sin(theta)*cos(phi) + sin(psi)*sin(phi);
            sin(psi)*cos(theta), sin(psi)*sin(theta)*sin(phi) + cos(psi)*cos(phi), sin(psi)*sin(theta)*cos(phi) - cos(psi)*sin(phi);
            -sin(theta),         cos(theta)*sin(phi),                            cos(theta)*cos(phi)];

    case 6     %inv(T)                                                            % Transformation from derivative of (phi theta psi) to body rates (p q r)
        rm = [ 1        0              -sin(theta)      ;
            0      cos(phi)     sin(phi)*cos(theta)  ;
            0     -sin(phi)     cos(phi)*cos(theta) ];

    case 7    %T                                                             % Transformation from body rates (p q r) to derivative of (phi theta psi)
        rm = [ 1, sin(phi)*tan(theta), cos(phi)*tan(theta);
            0, cos(phi), -sin(phi);
            0, sin(phi)/cos(theta), cos(phi)/cos(theta)];
    
    case 8    %transpose(R)                         % Transformation from inertial frame to body frame
        rm = [cos(psi)*cos(theta), sin(psi)*cos(theta), -sin(theta);
              cos(psi)*sin(theta)*sin(phi) - sin(psi)*cos(phi), sin(psi)*sin(theta)*sin(phi) + cos(psi)*cos(phi), cos(theta)*sin(phi);
              cos(psi)*sin(theta)*cos(phi) + sin(psi)*sin(phi), sin(psi)*sin(theta)*cos(phi) - cos(psi)*sin(phi), cos(theta)*cos(phi)];

end

end

== matlab function flight_data_collection/central difference ==
  data: p input; p_dot output; q input; r input; q_dot output; r_dot output
function [p_dot, q_dot, r_dot] = fcn(p, q, r)
    % 중앙 차분법으로 p_dot, q_dot, r_dot 계산
    % 그런데 중앙차분할때 미래의 데이터를 알아야하는데 알수가 없기 때문에 여기서 얻는 중앙차분값은 한스텦 이전의 상태에서의 미분값이다.

    % 상태 유지 변수
    persistent data_p data_q data_r dt initialized;

    % 초기화
    if isempty(initialized)
        data_p = zeros(3, 1); % 고정된 크기의 배열
        data_q = zeros(3, 1);
        data_r = zeros(3, 1);
        dt = 0.1; % 샘플링 간격
        initialized = true;
    end

    % FIFO 방식으로 데이터 업데이트
    data_p = [data_p(2:end); p]; % 가장 오래된 데이터 제거 후 새로운 데이터 추가
    data_q = [data_q(2:end); q];
    data_r = [data_r(2:end); r];

    % 중앙 차분법 적용 (배열 크기가 3인 경우)
    p_dot = (data_p(3) - data_p(1)) / (2 * dt); % 중앙 차분
    q_dot = (data_q(3) - data_q(1)) / (2 * dt); % 중앙 차분
    r_dot = (data_r(3) - data_r(1)) / (2 * dt); % 중앙 차분

    % disp("data_p = ");
    % disp(data_p);
end

== matlab function flight_data_collection/MotorForceCalculation/octo geometricCalc ==
  data: L1 input; C output; L2 input; L3 input; Ct input; Cq input; C_pseudo_inverse output
function [C,C_pseudo_inverse] = geometricCalc(L1,L2,L3,Ct,Cq)

% k= (1/sqrt(2));

% C : control matrix
% C+ : pseudo-inverse
% u* : pseudo input
% u : input
% u = C x u*

C = [ -Ct,  -Ct,  -Ct,  -Ct,  -Ct,  -Ct,  -Ct,  -Ct;
     -Ct*L1,  Ct*L1, -Ct*L1,  -Ct*L1,  Ct*L1, Ct*L1,  Ct*L1, -Ct*L1;
     Ct*L3,  -Ct*L3, Ct*L2,  -Ct*L3,  Ct*L3, -Ct*L2,  Ct*L2,  -Ct*L2;
      Cq,  Cq, -Cq, -Cq, -Cq, -Cq,  Cq,  Cq ];

C_pseudo_inverse = pinv(C);

% e = [ 0             -sin(alpha)     -cos(alpha);
%      -k*sin(alpha)  k*sin(alpha)    -cos(alpha);
%       sin(alpha)    0               -cos(alpha);
%      -k*sin(alpha)  -k*sin(alpha)   -cos(alpha);
%       0             sin(alpha)      -cos(alpha);
%       k*sin(alpha)  -k*sin(alpha)   -cos(alpha);
%      -sin(alpha)    0               -cos(alpha);
%       k*sin(alpha)  k*sin(alpha)    -cos(alpha)];
end

== matlab function flight_data_collection/MATLAB Function3 ==
  data: Central_M_B output; p_dot input; q_dot input; r_dot input; p input; q input; r input
function Central_M_B = fcn(p_dot,q_dot,r_dot,p,q,r)

% 한스텦 이전의 미분값 과 한스텦 이전의 상태 값을 이용하여 MB 계산

I_v = [1.52 0 0;0 7.47 0;0 0 8.89]; % octocopter

Central_M_B = I_v * [p_dot;q_dot;r_dot] + cross([p;q;r] , I_v * [p;q;r]);

== matlab function flight_data_collection/MotorForceCalculation/motorForceMomentCalc ==
  settings: updateMethod=DISCRETE
  data: omegaMotorSpeed input; FB output; MB output; C input
function [FB,MB] = motorForceMomentCalc(omegaMotorSpeed,C)

% FB = [fx; fy; fz];
% MB = [mx; my; mz];


% persistent 변수 선언
persistent is_initialized;

% 초기화가 필요할 때만 실행
if isempty(is_initialized)
    % 임시 변수에 초기화
    is_initialized = true;
end

FB_temp = zeros(3, 1);
MB_temp = zeros(3, 1);

% C : 4by8
% omegaMotor : 8by1
% actual_force_and_moment_acting_on_the_body = [ft; tau_x; tau_y; tau_z]'
actual_force_and_moment_acting_on_the_body = C * (abs(omegaMotorSpeed) .* abs(omegaMotorSpeed));
% actual_force_and_moment_acting_on_the_body = C * abs(omegaMotorSpeed);
% disp('omegaMotor = ')
% disp(abs(omegaMotorSpeed))
% disp('omegaMotor.^2 = ')
% disp(abs(omegaMotorSpeed) .* abs(omegaMotorSpeed))

FB_temp(1) = 0;
FB_temp(2) = 0;
FB_temp(3) = actual_force_and_moment_acting_on_the_body(1); % 추력 (Thrust)
MB_temp(1) = actual_force_and_moment_acting_on_the_body(2); % 롤 모멘트 (Roll moment)
MB_temp(2) = -actual_force_and_moment_acting_on_the_body(3); % 피치 모멘트 (Pitch moment)
MB_temp(3) = -actual_force_and_moment_acting_on_the_body(4); % 요 모멘트 (Yaw moment)

% 계산 결과를 출력 변수에 할당
FB = FB_temp;
MB = MB_temp;


end

== matlab function flight_data_collection/MATLAB Function ==
  data: backward_M_B output; p_dot input; q_dot input; r_dot input; p input; q input; r input
function backward_M_B = fcn(p_dot,q_dot,r_dot,p,q,r)


I_v = [1.52 0 0;0 7.47 0;0 0 8.89]; % octocopter

backward_M_B = I_v * [p_dot;q_dot;r_dot] + cross([p;q;r] , I_v * [p;q;r]);
